simulink model "part_one"  (R2019b)
settings: Solver=VariableStepAuto  StartTime=0.0  StopTime=10.0  RelTol=1e-3
settings Model: Creator=adityaaaap  LastModifiedBy=adityaaaap
settings DataIOCC: ReturnWorkspaceOutputs=off
settings DebuggingCC: ArithmeticOperatorsInVariantConditions=warning
settings SFSimCC: SimUseLocalCustomCode=off  CustomCodeUndefinedFunction=UseInterfaceOnly
settings RTWCC: RTWUseLocalCustomCode=off
settings CodeAppCC: StateflowObjectComments=on

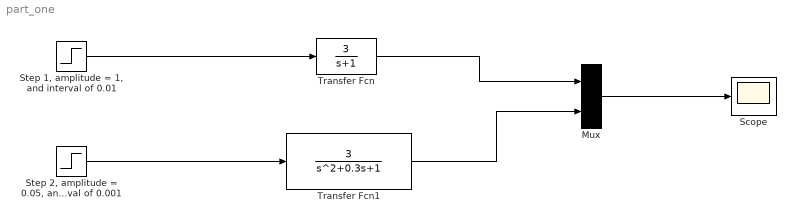
== system part_one ==
  Mux : Mux  Inputs=2
  Scope : Scope
  "Step 1, amplitude = 1, and interval of 0.01" : Step  Time=0  SampleTime=0.01
  "Step 2, amplitude = 0.05, and interval of 0.001 " : Step  Time=0  After=0.5  SampleTime=0.001
  Transfer Fcn : TransferFcn  Numerator=[3]  Denominator=[1 1]
  Transfer Fcn1 : TransferFcn  Numerator=[3]  Denominator=[1 0.3 1]
  wires:
  "Step 1, amplitude = 1, and interval of 0.01"/1 -> Transfer Fcn/1
  Transfer Fcn/1 -> Mux/1
  Transfer Fcn1/1 -> Mux/2
  "Step 2, amplitude = 0.05, and interval of 0.001 "/1 -> Transfer Fcn1/1
  Mux/1 -> Scope/1
